simulink model "grid_ups"  (R2024b)
settings: Solver=VariableStepAuto  StartTime=0.0  StopTime=0.2  RelTol=1e-3
undefined symbols (not defined in the file): Ion, Lithium
libraries: spsIGBTDiodeLib x4, spsDiodeLib x4, spsCurrentMeasurementLib x2, spsVoltageMeasurementLib x2, spsACVoltageSourceLib x1, spsBatteryLib x1, spsBreakerLib x1, spsTriangleGeneratorLib x1, spsSeriesRLCBranchLib x1, sps_lib x1
settings Model: Creator=rushi  LastModifiedBy=rushi
settings DataIOCC: ReturnWorkspaceOutputs=off

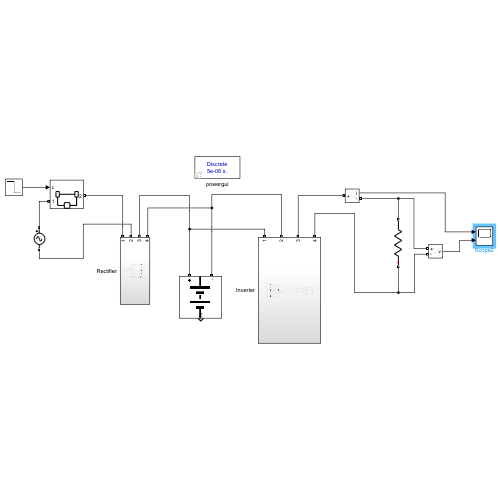
[thumbnail: Simulink's stored preview of the top-level diagram]
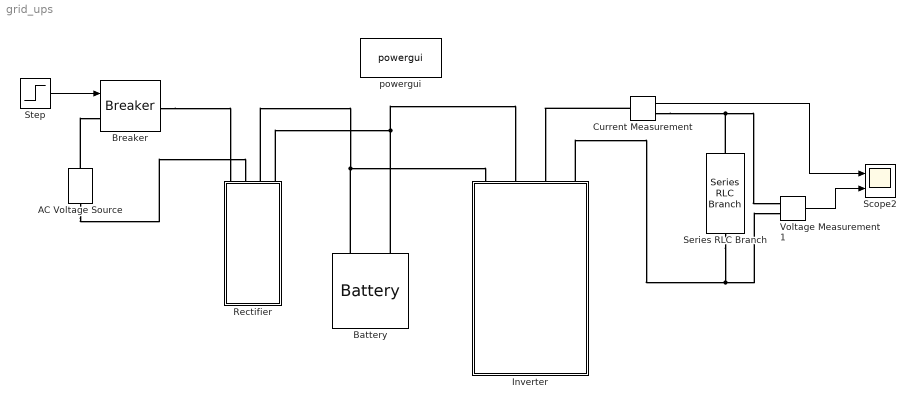
== system grid_ups ==
  AC Voltage Source : spsACVoltageSourceLib/AC Voltage Source  Amplitude=100  Phase=0  Frequency=50  SampleTime=0  Measurements=None  BusType=swing  Pref=10e3  Qref=0  Qmin=-inf  Qmax=+inf
  Battery : spsBatteryLib/Battery  BatType=Lithium-Ion  NomV=86  NomQ=100  SOC=100  Batt_Tr=600  PresetModel=on  MaxQ=100  MinV=64.5  FullV=100.1029  Dis_rate=43.4783  R=0.0086  Normal_OP=90.4348  expZone="[92.9132      4.91304]"
  Breaker : spsBreakerLib/Breaker  InitialState=1  SwitchingTimes="[1/60  5/60]"  External=on  BreakerResistance=0.01  SnubberResistance=1e6  SnubberCapacitance=inf  Measurements=None  MoreParameters=on  NoBreakLoop=off
  Current Measurement : spsCurrentMeasurementLib/Current Measurement  PhasorSimulation=off  OutputType=Complex  PSBequivalent=0
  Inverter : Subsystem
  Rectifier : Subsystem
  Scope2 : Scope  NumInputPorts=2
  Series RLC Branch : spsSeriesRLCBranchLib/Series RLC Branch  LConnTagsString=__new0  RConnTagsString=__new0  BranchType=R  Resistance=1  Inductance=1e-3  SetiL0=off  InitialCurrent=0  Capacitance=1e-6  Setx0=off  InitialVoltage=0  Measurements=None
  Step : Step  Time=0.5  Before=1  After=0  SampleTime=0
  Voltage Measurement1 : spsVoltageMeasurementLib/Voltage Measurement  PhasorSimulation=off  OutputType=Complex  PSBequivalent=0
  powergui : sps_lib/powergui  Priority=1  SimulationMode=Discrete  SampleTime=5e-6  frequency=60  Iterations=50  frequencyindice=0  Pbase=100e6  ErrMax=1e-4  UnitsV=kV  UnitsW=MW  buscounter=0  FunctionMessages=off  echomessages=off  EnableUseOfTLC=off  CurrentSourceSwitches=off  DisableSnubberDevices=off  DisableRonSwitches=off  DisableVfSwitches=off  DisplayEquations=off  AutomaticDiscreteSolvers=off  SolverType=Tustin/Backward Euler (TBE)  Interpol=off  ExternalGateDelay=off  methode=off  Ts=100  x0status=blocks  SPID=on  SwTol=0  HookPort=off  NonlinearTolerance=1e-4  nMaxIteration=100  ContinueOnMaxIteration=off  RestoreLinks=warning  ResistiveCurrentMeasurement=off  Frange=[0:2:500]  Ylog=off  Xlog=on  ShowGrid=off  save=off  variable=ZData  structure=0  ZoomFFT=off  StartTime=0.0  cycles=1  DisplayStyle=1  fundamental=60  FreqAxis=off  MaxFrequency=1000  frequencyindicesteady=1  RmsSteady=1  display=off
  wires:
  Step/1 -> Breaker/1
  Voltage Measurement1/1 -> Scope2/2
  Current Measurement/1 -> Scope2/1
  connections:
  Series RLC Branch/RConn1 -- Current Measurement/RConn1 -- Voltage Measurement1/LConn1
  Series RLC Branch/LConn1 -- Inverter/LConn4 -- Voltage Measurement1/LConn2
  AC Voltage Source/RConn1 -- Breaker/LConn1
  Current Measurement/LConn1 -- Inverter/LConn3
  Battery/LConn1 -- Rectifier/LConn3 -- Inverter/LConn1
  Battery/LConn2 -- Rectifier/LConn4 -- Inverter/LConn2
  Breaker/RConn1 -- Rectifier/LConn1
  AC Voltage Source/LConn1 -- Rectifier/LConn2

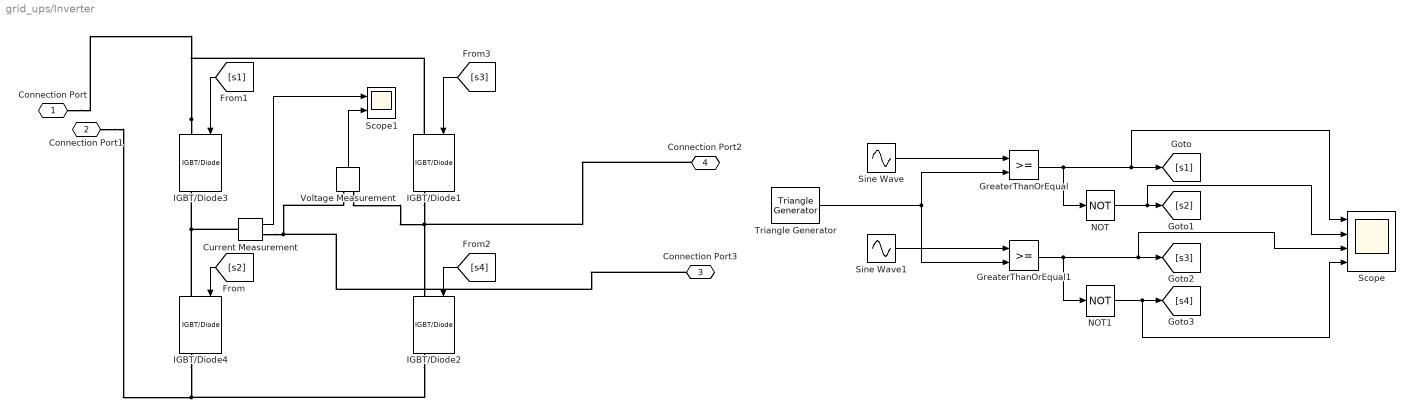
== system grid_ups/Inverter ==
  Current Measurement : spsCurrentMeasurementLib/Current Measurement  PhasorSimulation=off  OutputType=Complex  PSBequivalent=0
  GreaterThanOrEqual : RelationalOperator  OutDataTypeStr=boolean  RndMeth=Simplest  InputSameDT=off
  GreaterThanOrEqual1 : RelationalOperator  OutDataTypeStr=boolean  RndMeth=Simplest  InputSameDT=off
  IGBT/Diode{1..4} (4 alike) : spsIGBTDiodeLib/IGBT//Diode  Ron=1e-3  Rs=1e5  Cs=inf  Measurements=on
  NOT : Logic  Operator=NOT  IconShape=distinctive  AllPortsSameDT=off  OutDataTypeStr=boolean
  NOT1 : Logic  Operator=NOT  IconShape=distinctive  AllPortsSameDT=off  OutDataTypeStr=boolean
  Scope : Scope  NumInputPorts=4
  Scope1 : Scope  NumInputPorts=2
  Sine Wave : Sin  Frequency=2*pi*50  SampleTime=0
  Sine Wave1 : Sin  Frequency=2*pi*50  Phase=pi  SampleTime=0
  Triangle Generator : spsTriangleGeneratorLib/Triangle Generator  Freq=2000  Phase=0  Ts=0
  Voltage Measurement : spsVoltageMeasurementLib/Voltage Measurement  PhasorSimulation=off  OutputType=Complex  PSBequivalent=0
  Connection Port : PMIOPort  Side=Left
  Connection Port1 : PMIOPort  Port=2  Side=Left
  Connection Port3 : PMIOPort  Port=3  Side=Left
  Connection Port2 : PMIOPort  Port=4  Side=Left
  wires:
  [s2] -> IGBT/Diode4/1
  [s1] -> IGBT/Diode3/1
  [s4] -> IGBT/Diode2/1
  Current Measurement/1 -> Scope1/1
  Voltage Measurement/1 -> Scope1/2
  [s3] -> IGBT/Diode1/1
  GreaterThanOrEqual/1 -> Scope/1, [s1], NOT/1
  GreaterThanOrEqual1/1 -> NOT1/1, Scope/3, [s3]
  Sine Wave1/1 -> GreaterThanOrEqual1/1
  Triangle Generator/1 -> GreaterThanOrEqual1/2, GreaterThanOrEqual/2
  Sine Wave/1 -> GreaterThanOrEqual/1
  NOT1/1 -> Scope/4, [s4]
  NOT/1 -> Scope/2, [s2]
  connections:
  IGBT/Diode4/RConn1 -- Connection Port1/RConn1 -- IGBT/Diode2/RConn1
  IGBT/Diode1/RConn1 -- Connection Port2/RConn1 -- IGBT/Diode2/LConn1 -- Voltage Measurement/LConn2
  Current Measurement/LConn1 -- IGBT/Diode4/LConn1 -- IGBT/Diode3/RConn1
  Voltage Measurement/LConn1 -- Connection Port3/RConn1 -- Current Measurement/RConn1
  IGBT/Diode3/LConn1 -- Connection Port/RConn1 -- IGBT/Diode1/LConn1

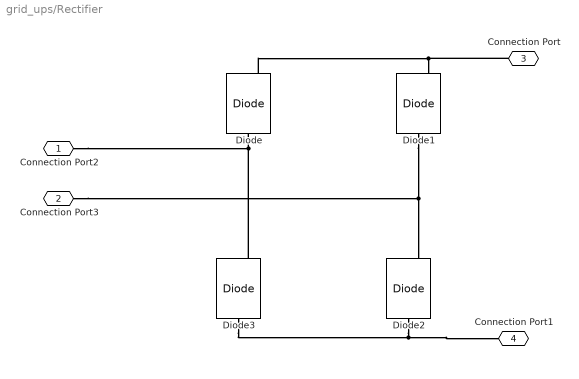
== system grid_ups/Rectifier ==
  Diode{,1..3} (4 alike) : spsDiodeLib/Diode  Ron=0.001  Lon=0  Vf=0.8  IC=0  UseSnubber=0  Rs=500  Cs=250e-9  Measurements=on
  Connection Port2 : PMIOPort  Side=Left
  Connection Port3 : PMIOPort  Port=2  Side=Left
  Connection Port : PMIOPort  Port=3  Side=Left
  Connection Port1 : PMIOPort  Port=4  Side=Left
  connections:
  Diode3/RConn1 -- Connection Port2/RConn1 -- Diode/LConn1
  Diode1/LConn1 -- Diode2/RConn1 -- Connection Port3/RConn1
  Diode1/RConn1 -- Connection Port/RConn1 -- Diode/RConn1
  Diode3/LConn1 -- Diode2/LConn1 -- Connection Port1/RConn1
